simulink model "RALFWinkel17b"  (R2018b)
settings: Solver=FixedStepAuto  StartTime=0.0  StopTime=inf  FixedStep=0.01  RelTol=1e-3  EnableMultiTasking=on
libraries: robotlib x4, simulink x2, sensehatlib x1
settings Model: SimulationMode=external  ExtModeTrigDuration=10000  ExtModeArchiveMode=auto  ExtModeArchiveFileName=testlog  ExtModeArchiveDirName=/home/alf/Matlab/RALF  Creator=alf  LastModifiedBy=HannesDittmann
settings SolverCC: PositivePriorityOrder=on
settings DataIOCC: LoggingToFile=on
settings OptimizationCC: PassReuseOutputArgsAs=Individual arguments  MaxStackSize=64
settings DebuggingCC: ParameterTunabilityLossMsg=error
settings HardwareCC: ProdBitPerPointer=32  ProdBitPerSizeT=32  ProdBitPerPtrDiffT=32  ProdLargestAtomicInteger=Long  ProdLargestAtomicFloat=Double  ProdWordSize=32  ProdHWDeviceType=ARM Compatible->ARM Cortex
settings SFSimCC: SimUseLocalCustomCode=off  MATLABDynamicMemAlloc=off
settings RTWCC: SystemTargetFile=ert.tlc  HardwareBoard=Raspberry Pi - Robot Operating System (ROS)  TLCOptions="-aInlineSetEventsForThisBaseRateFcn=TLC_FALSE -aSuppressMultiTaskScheduler=TLC_FALSE  -aRateBasedStepFcn=0"  TemplateMakefile=ert_default_tmf  GenerateReport=on  RTWUseLocalCustomCode=off  Toolchain=Catkin  IncludeHyperlinkInReport=on  LaunchReport=on  TargetLang=C++  GenerateTraceInfo=on  GenerateTraceReport=on  GenerateTraceReportSl=on  GenerateTraceReportSf=on  GenerateTraceReportEml=on
settings CodeAppCC: ForceParamTrailComments=on  IgnoreCustomStorageClasses=off  OperatorAnnotations=on  SimulinkDataObjDesc=on  SFDataObjDesc=on  InsertBlockDesc=on
settings ERTTargetCC: SupportContinuousTime=on  SupportVariableSizeSignals=on  ExtMode=on

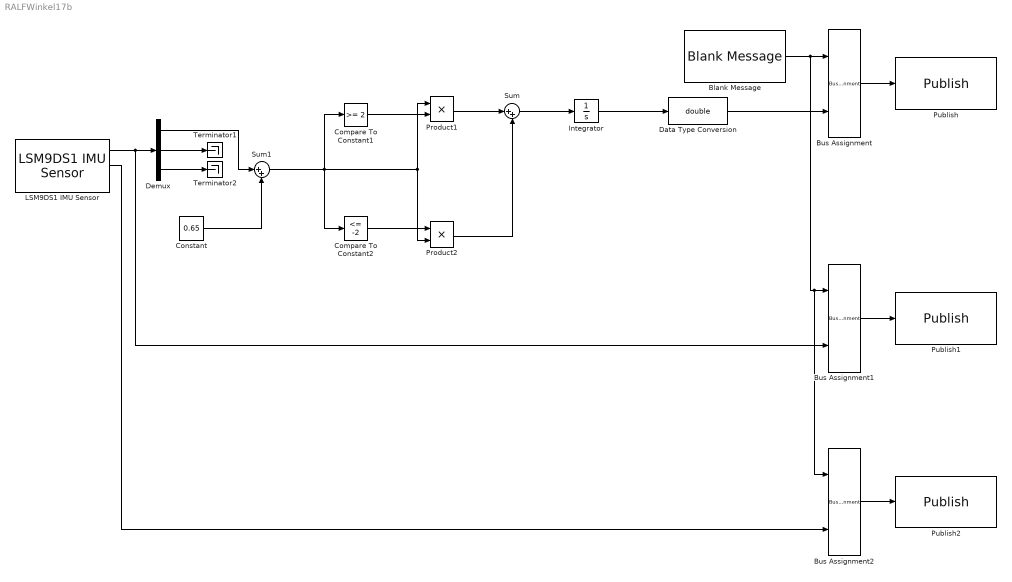
== system RALFWinkel17b ==
  Blank Message : robotlib/Blank Message  messageClass=Message  entityType=geometry_msgs/Point  messageType=geometry_msgs/Point  SampleTime=inf
      settings: SourceProductBaseCode=RO
  Bus Assignment : BusAssignment  AssignedSignals=Z
  Bus Assignment1 : BusAssignment  AssignedSignals=Z
  Bus Assignment2 : BusAssignment  AssignedSignals=Z
  Compare To Constant1 : simulink/Logic and Bit Operations/Compare To Constant  relop=>=  const=2  OutDataTypeStr=boolean
  Compare To Constant2 : simulink/Logic and Bit Operations/Compare To Constant  relop=<=  const=-2  OutDataTypeStr=boolean
  Constant : Constant  Value=0.65
  Data Type Conversion : DataTypeConversion  OutDataTypeStr=double
  Demux : Demux  Outputs=3
  Integrator : Integrator
  LSM9DS1 IMU Sensor : sensehatlib/LSM9DS1 IMU Sensor  blockPlatform=Raspberry Pi  BoardProperty_sh=Pi 2 Model B  ActiveSensors_=Accelerometer, Gyroscope and Magnetometer  AccelerometerOutputDataRate=119 Hz  AccelerometerFullScaleRange=+/- 2g  AccelerometerBandwidth=50 Hz  GyroscopeOutputDataRate=119 Hz  GyroscopeFullScaleRange=245 dps  GyroscopeBandwidthMode=0  GyroscopeHighPassFilterEnabled=off  GyroscopeHighPassFilterMode=0  MagnetometerFullScaleRange=+/- 4 gauss  MagnetometerOutputDataRate=40 Hz  SampleTime=0.01
      settings: SourceProductName=Simulink Support Package for Raspberry Pi Hardware  SourceProductBaseCode=RASPPI
  Product1 : Product
  Product2 : Product
  Publish : robotlib/Publish  topicSource=Specify your own  topic=/ralfwinkel  messageType=geometry_msgs/Point  messageQueueLength=1
      settings: SourceProductBaseCode=RO
  Publish1 : robotlib/Publish  topicSource=Specify your own  topic=/ralfAngVel  messageType=geometry_msgs/Point  messageQueueLength=1
      settings: SourceProductBaseCode=RO
  Publish2 : robotlib/Publish  topicSource=Specify your own  topic=/ralfAccel  messageType=geometry_msgs/Point  messageQueueLength=1
      settings: SourceProductBaseCode=RO
  Sum : Sum  Inputs=|++
  Sum1 : Sum  Inputs=|++
  Terminator1 : Terminator
  Terminator2 : Terminator
  wires:
  Product1/1 -> Sum/1
  Product2/1 -> Sum/2
  Compare To Constant1/1 -> Product1/2
  Compare To Constant2/1 -> Product2/1
  LSM9DS1 IMU Sensor/1 -> Bus Assignment1/2, Demux/1
  Sum/1 -> Integrator/1
  Integrator/1 -> Data Type Conversion/1
  Constant/1 -> Sum1/2
  Sum1/1 -> Compare To Constant2/1, Product2/2, Product1/1, Compare To Constant1/1
  Demux/1 -> Sum1/1
  Demux/2 -> Terminator1/1
  Blank Message/1 -> Bus Assignment2/1, Bus Assignment1/1, Bus Assignment/1
  Bus Assignment/1 -> Publish/1
  Data Type Conversion/1 -> Bus Assignment/2
  Demux/3 -> Terminator2/1
  Bus Assignment1/1 -> Publish1/1
  Bus Assignment2/1 -> Publish2/1
  LSM9DS1 IMU Sensor/2 -> Bus Assignment2/2
